simulink model "plc"  (R2023a)
settings: Solver=VariableStepAuto  StartTime=0.0  StopTime=inf  RelTol=1e-3
undefined symbols (not defined in the file): a1, A1, g, H1_max, Q1_max, s12
libraries: dspnetwork x3
settings Model: Creator=Dottorandi  LastModifiedBy=Francesco
settings SolverCC: AlgebraicLoopSolver=TrustRegion
settings DataIOCC: ReturnWorkspaceOutputs=off
settings DebuggingCC: UnconnectedInputMsg=warning  UnconnectedOutputMsg=warning  UnconnectedLineMsg=warning  ArithmeticOperatorsInVariantConditions=warning
settings ModelReferenceCC: EnableRefExpFcnMdlSchedulingChecks=on
settings SFSimCC: SimUseLocalCustomCode=off  CustomCodeUndefinedFunction=UseInterfaceOnly
settings RTWCC: RTWUseLocalCustomCode=off  DLArmComputeVersion=19.05

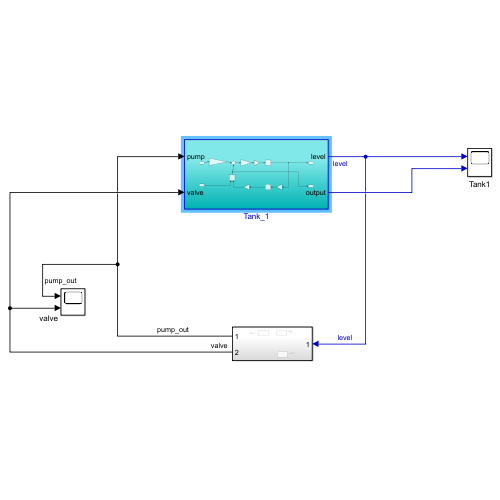
[thumbnail: Simulink's stored preview of the top-level diagram]
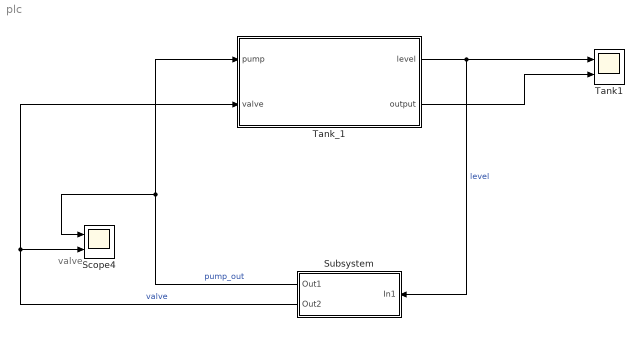
== system plc ==
  note: valve
  Scope4 : Scope  NumInputPorts=2
  Subsystem : Subsystem
  Tank1 : Scope  NumInputPorts=2
  Tank_1 : Subsystem
  wires:
  Tank_1/1(level) -> Subsystem/1(In1), Tank1/1  "level"
  Tank_1/2(output) -> Tank1/2
  Subsystem/2(Out2) -> Scope4/2, Tank_1/2(valve)  "valve"
  Subsystem/1(Out1) -> Scope4/1, Tank_1/1(pump)  "pump_out"

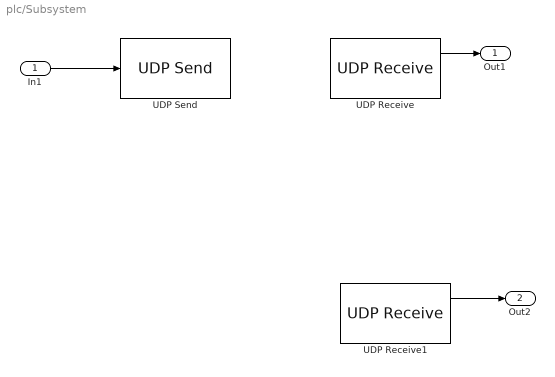
== system plc/Subsystem ==
  In1 : Inport
  UDP Receive : dspnetwork/UDP Receive  localURL='0.0.0.0'  localPort=10012  remoteURL='0.0.0.0'  remotePort=-1  recvBufferSize=2  dims=1  signalDatatype=uint16  isComplex=off  isVarSize=off  showBlockingTime=on  blockingTime=0  sampletime=1  blockPlatform=LINUX
  UDP Receive1 : dspnetwork/UDP Receive  localURL='0.0.0.0'  localPort=10013  remoteURL='0.0.0.0'  remotePort=-1  recvBufferSize=2  dims=1  signalDatatype=uint16  isComplex=off  isVarSize=off  showBlockingTime=on  blockingTime=0  sampletime=1  blockPlatform=LINUX
  UDP Send : dspnetwork/UDP Send  remoteURL='127.0.0.1'  remotePort=10001  localURL='255.255.255.255'  localPortSource=Automatically determine  localPort=-1  sendBufferSize=8192  sampletime=-1  blockPlatform=LINUX  separateLengthPort=0
  Out1 : Outport  VectorParamsAs1DForOutWhenUnconnected=off
  Out2 : Outport  Port=2  VectorParamsAs1DForOutWhenUnconnected=off
  wires:
  In1/1 -> UDP Send/1
  UDP Receive/1 -> Out1/1
  UDP Receive1/1 -> Out2/1

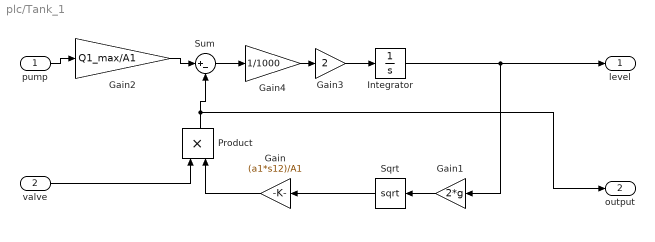
== system plc/Tank_1 ==
  pump : Inport
  valve : Inport  Port=2
  Gain : Gain  Gain=(a1*s12)/A1
  Gain1 : Gain  Gain=2*g
  Gain2 : Gain  Gain=Q1_max/A1
  Gain3 : Gain  Gain=2
  Gain4 : Gain  Gain=1/1000
  Integrator : Integrator  InitialCondition=0.11*H1_max  LimitOutput=on  UpperSaturationLimit=100  LowerSaturationLimit=0
  Product : Product
  Sqrt : Sqrt
  Sum : Sum  Inputs=|+-
  level : Outport  VectorParamsAs1DForOutWhenUnconnected=off
  output : Outport  Port=2  VectorParamsAs1DForOutWhenUnconnected=off
  wires:
  pump/1 -> Gain2/1
  Integrator/1 -> Gain1/1, level/1
  Sum/1 -> Gain4/1
  Gain/1 -> Product/2
  Sqrt/1 -> Gain/1
  Gain1/1 -> Sqrt/1
  valve/1 -> Product/1
  Product/1 -> output/1, Sum/2
  Gain2/1 -> Sum/1
  Gain3/1 -> Integrator/1
  Gain4/1 -> Gain3/1
